simulink model "pendulum"  (R2023b)
settings: Solver=VariableStepAuto  StartTime=0.0  StopTime=60  RelTol=1e-3
settings Model: Creator=mateisorodoc  LastModifiedBy=mateisorodoc

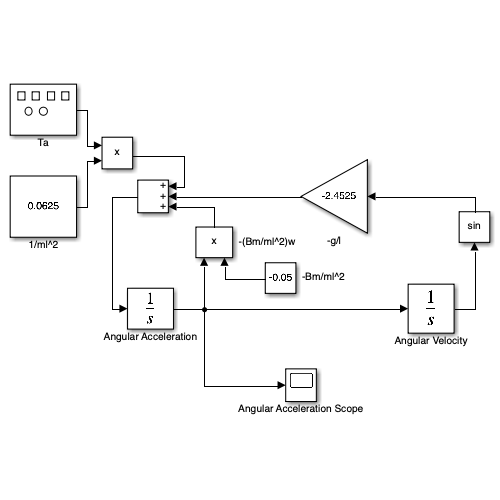
[thumbnail: Simulink's stored preview of the top-level diagram]
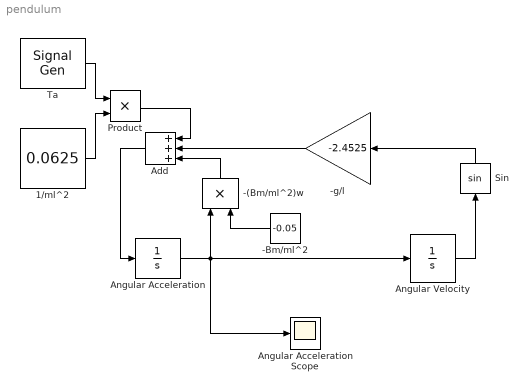
== system pendulum ==
  -(Bm/ml^2)w : Product
  -Bm/ml^2 : Constant  Value=-0.05
  -g/l : Gain  Gain=-2.4525
  1/ml^2 : Constant  Value=0.0625
  Add : Sum  Inputs=+++
  Angular Acceleration : Integrator
  Angular Acceleration Scope : Scope
  Angular Velocity : Integrator
  Product : Product
  Sin : Trigonometry
  Ta : SignalGenerator  WaveForm=sawtooth  Frequency=0.1  Units=rad/sec
  wires:
  Angular Velocity/1 -> Sin/1
  Sin/1 -> -g/l/1
  Ta/1 -> Product/1
  1/ml^2/1 -> Product/2
  Product/1 -> Add/1
  -g/l/1 -> Add/2
  Add/1 -> Angular Acceleration/1
  -Bm/ml^2/1 -> -(Bm/ml^2)w/2
  -(Bm/ml^2)w/1 -> Add/3
  Angular Acceleration/1 -> Angular Acceleration Scope/1, Angular Velocity/1, -(Bm/ml^2)w/1
